simulink model "lab5p2pid (conflict)"  (R2020a)
settings: Solver=FixedStepAuto  StartTime=0.0  StopTime=2.2  FixedStep=0.005/15  RelTol=1e-3
libraries: roblocks x6
settings Model: Creator=assetmalik  LastModifiedBy=assetmalik

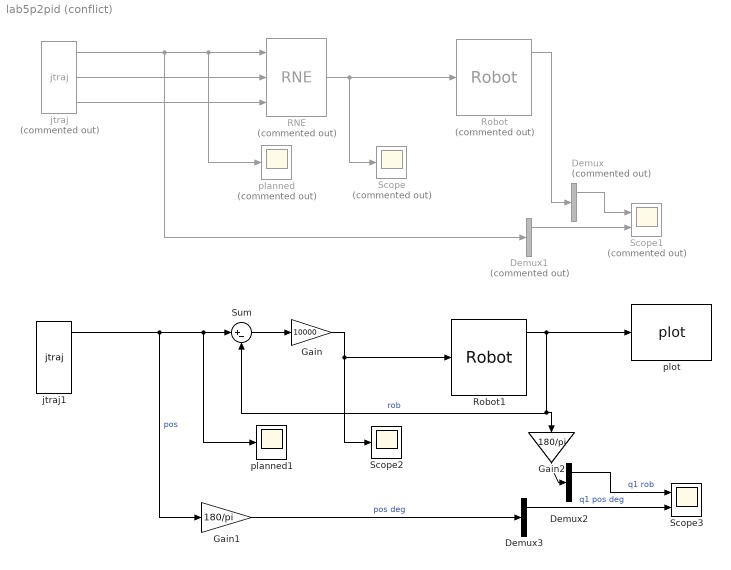
== system lab5p2pid (conflict) ==
  Demux : Demux  Commented=on  Outputs=3
  Demux1 : Demux  Commented=on  Outputs=3
  Demux2 : Demux  Outputs=3
  Demux3 : Demux  Outputs=3
  Gain : Gain  Gain=10000
  Gain1 : Gain  Gain=180/pi
  Gain2 : Gain  Gain=180/pi
  RNE : roblocks/Arm/RNE  Commented=on  robot=theRb_l5  grav=[0 0 9.81]
  Robot : roblocks/Arm/Robot  Commented=on  robot=theRb_l5  q0=[0 0 0]
  Robot1 : roblocks/Arm/Robot  robot=theRb_l5  q0=[0 0 0]
  Scope : Scope  Commented=on
  Scope1 : Scope  Commented=on  NumInputPorts=2
  Scope2 : Scope
  Scope3 : Scope  NumInputPorts=2
  Sum : Sum  Inputs=|+-
  jtraj : roblocks/Toolbox/jtraj  Commented=on  q0=[0 0 0]  qf=[pi/2 -pi/4 -pi/4]  tmax=2  ts=0.005
  jtraj1 : roblocks/Toolbox/jtraj  q0=[0 0 0]  qf=[pi/2 -pi/4 -pi/4]  tmax=2  ts=0.005
  planned : Scope  Commented=on
  planned1 : Scope
  plot : roblocks/Arm/plot  robot=theRb_l5  fps=15  holdplot=on
  wires:
  jtraj/1 -> Demux1/1, planned/1, RNE/1
  RNE/1 -> Scope/1, Robot/1
  jtraj/2 -> RNE/2
  jtraj/3 -> RNE/3
  Robot/1 -> Demux/1
  Demux/1 -> Scope1/1
  Demux1/1 -> Scope1/2
  Gain/1 -> Scope2/1, Robot1/1
  Robot1/1 -> plot/1, Gain2/1, Sum/2  "rob"
  Demux2/1 -> Scope3/1  "q1 rob"
  Demux3/1 -> Scope3/2  "q1 pos deg"
  jtraj1/1 -> Gain1/1, Sum/1, planned1/1  "pos"
  Gain1/1 -> Demux3/1  "pos deg"
  Sum/1 -> Gain/1
  Gain2/1 -> Demux2/1
